simulink model "laba2"  (R2017a)
settings: Solver=VariableStepAuto  StartTime=0.0  StopTime=30  MaxStep=0.01  RelTol=1e-3
libraries: simulink x1
settings Model: Creator=alanik99  LastModifiedBy=alanik99

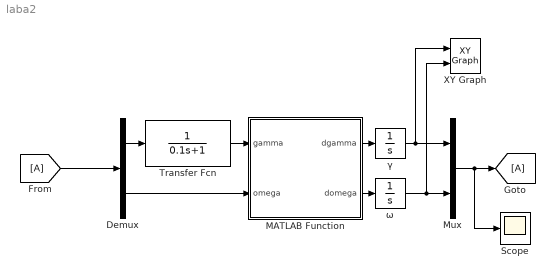
== system laba2 ==
  Demux : Demux  Outputs=2
  MATLAB Function : MATLAB Function  TreatAsAtomicUnit=on
  Mux : Mux  Inputs=2
  Scope : Scope
  Transfer Fcn : TransferFcn  Denominator=[0.1 1]
  XY Graph : simulink/Sinks/XY Graph  xmin=-7  xmax=21  ymin=-21  ymax=17  st=-1
  γ : Integrator  InitialCondition=20
  ω : Integrator  InitialCondition=-0.0000001
  wires:
  [A] -> Demux/1
  Demux/2 -> MATLAB Function/2(omega)
  MATLAB Function/1(dgamma) -> γ/1
  MATLAB Function/2(domega) -> ω/1
  γ/1 -> XY Graph/1, Mux/1
  ω/1 -> XY Graph/2, Mux/2
  Mux/1 -> Scope/1, [A]
  Demux/1 -> Transfer Fcn/1
  Transfer Fcn/1 -> MATLAB Function/1(gamma)

== matlab function laba2/MATLAB Function ==
  data: gamma input; dgamma output; omega input; domega output
function [dgamma, domega] = fcn(gamma, omega)

%% Задача 1 и Задача 4
c22 = -1.9;
c23 = 3.9;
deltaPre = 10;


if gamma > 0
    v = 1;
elseif gamma < 0
    v = -1;
else
    v = 0;
end

dgamma = omega;
domega = c22 * omega - c23 * deltaPre * v;

%% Задача 2
% c22 = -1.9;
% c23 = 3.9;
% 
% i1 = 1;
% i2 = 1;
% deltaPre = 10;
% e0 = 2;
% 
% if (gamma > e0/i1 && omega > 0) || (gamma > -e0/i1 && omega < 0)
%     v = 1;
% elseif (gamma < e0/i1 && omega > 0) || (gamma < -e0/i1 && omega < 0)
%     v = -1;
% else
%     v = 0;
% end
% 
% dgamma = omega;
% domega = c22 * omega - c23 * deltaPre * v;

%% Задача 3
% c22 = -1.9;
% c23 = 3.9;
% 
% i1 = 1;
% i2 = 1;
% deltaPre = 10;
% e0 = 2;
% 
% e = i1*gamma + i2*omega;
% 
% if (e > e0 && omega > 0) || (e > -e0 && omega < 0)
%     v = 1;
% elseif (e < e0 && omega > 0) || (e < -e0 && omega < 0)
%     v = -1;
% else
%     v = 0;
% end
% 
% dgamma = omega;
% domega = c22 * omega - c23 * deltaPre * v;
